simulink model "hw2p2f"  (R2017a)
settings: Solver=FixedStepAuto  StartTime=0.0  StopTime=10.0  FixedStep=0.1  RelTol=1e-3
libraries: powerlib_meascontrol x1
settings Model: Creator=Soutrik  LastModifiedBy=Soutrik

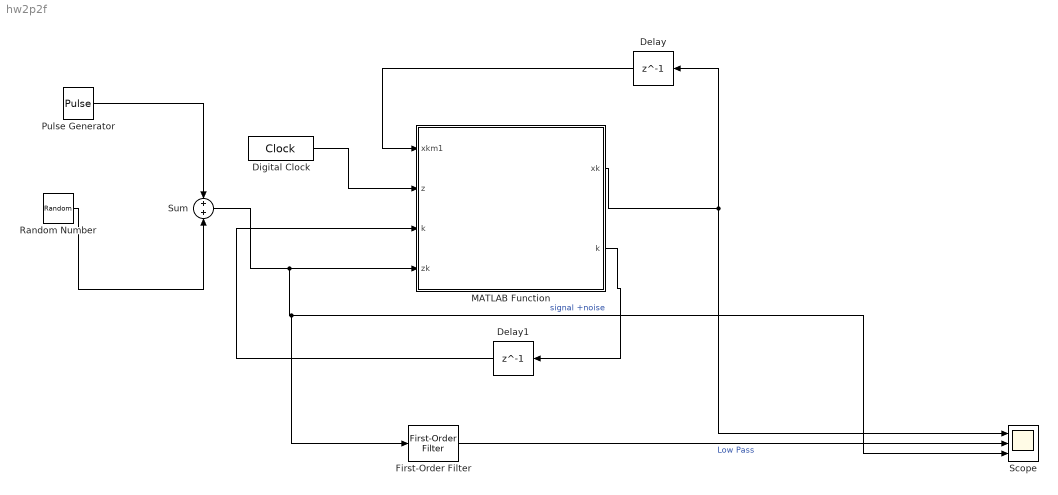
== system hw2p2f ==
  Delay : Delay  DelayLength=1  InitialCondition=0  SampleTime=0.1
  Delay1 : Delay  DelayLength=1  InitialCondition=0  SampleTime=0.1
  Digital Clock : DigitalClock  SampleTime=0.1
  First-Order Filter : powerlib_meascontrol/Filters/First-Order Filter  FilterType=Lowpass  Tc=9  Ts=0.1  Initialize=on  Vac_Init=[0, 0, 60]  Vdc_Init=0  PlotResponse=off  FreqRange="[0,  200,  1]"
      settings: SourceProductName=Simscape Power Systems
  MATLAB Function : MATLAB Function  TreatAsAtomicUnit=on
  Pulse Generator : DiscretePulseGenerator  PulseType=Time based  Period=5  PulseWidth=50
  Random Number : RandomNumber  Variance=0.005  SampleTime=0.1
  Scope : Scope  NumInputPorts=3
  Sum : Sum
  wires:
  Pulse Generator/1 -> Sum/1
  Random Number/1 -> Sum/2
  MATLAB Function/1(xk) -> Delay/1, Scope/1
  Delay/1 -> MATLAB Function/1(xkm1)
  MATLAB Function/2(k) -> Delay1/1
  Digital Clock/1 -> MATLAB Function/2(z)
  Delay1/1 -> MATLAB Function/3("k ")
  Sum/1 -> First-Order Filter/1, Scope/3, MATLAB Function/4(zk)  "signal +noise"
  First-Order Filter/1 -> Scope/2  "Low Pass"

== matlab function hw2p2f/MATLAB Function ==
  data: xkm1 input; z input; k input; xk output; zk input; k output
function [xk,k]= fcn(xkm1,z,k,zk)

  if z< 0.2
      k=1;
  else
      k=k+1;
  end
  
  if k>1
      k=1;
  end

  xk=xkm1+(1/(k))*(zk-xkm1);
